simulink model "simulationObservateur"  (R2015a)
settings: Solver=ode45  StartTime=0.0  StopTime=10.0  RelTol=1e-3
undefined symbols (not defined in the file or in its folder): EE2, obsv
settings Model: Creator=Lucien  LastModifiedBy=Lucien

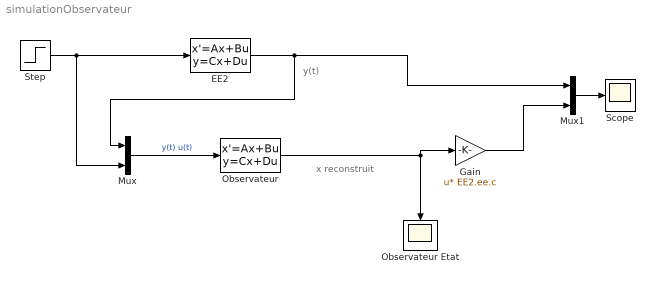
== system simulationObservateur ==
  note: x reconstruit
  note: y(t)
  "EE2 " : StateSpace  A=EE2.ee.a  B=EE2.ee.b  C=EE2.ee.c  D=EE2.ee.d  X0=0
  Gain : Gain  Gain=EE2.ee.c  Multiplication=Matrix(u*K)
  Mux : Mux  Inputs=2
  Mux1 : Mux  Inputs=2
  "Observateur " : StateSpace  A=obsv.ee.a  B=obsv.ee.b  C=obsv.ee.c  D=obsv.ee.d  X0=0
  "Observateur Etat " : Scope
  Scope : Scope
  Step : Step  Time=0  SampleTime=0
  wires:
  Mux/1 -> "Observateur "/1  "y(t) u(t)"
  "EE2 "/1 -> Mux1/1, Mux/1
  Mux1/1 -> Scope/1
  Step/1 -> Mux/2, "EE2 "/1
  Gain/1 -> Mux1/2
  "Observateur "/1 -> "Observateur Etat "/1, Gain/1
